simulink model "IM_Model"  (R2021a)
settings: Solver=ode23t  StartTime=0.0  StopTime=2  MaxStep=10^-5  RelTol=1e-3
InitFcn:
  | Rs=0.5968;
  | Lls=0.0003495;
  | Rr=0.6258;
  | Llr=0.005473;
  | Lm=0.0354;
  | Ls=Lls+Lm;
  | Lr=Llr+Lm;
  | J=0.05;
  | B=0.005879;
  | P=4;
libraries: spsControlledVoltageSourceLib x3, spsdq0toabcLib x2, spsAsynchronousMachineSIUnitsLib x1, mcbcontrolslib x1, spsabctodq0Lib x1, spspowerguiLib x1
settings Model: Creator=User  LastModifiedBy=User
settings SolverCC: AlgebraicLoopSolver=TrustRegion
settings DebuggingCC: SFMachineParentedDataDiag=warning

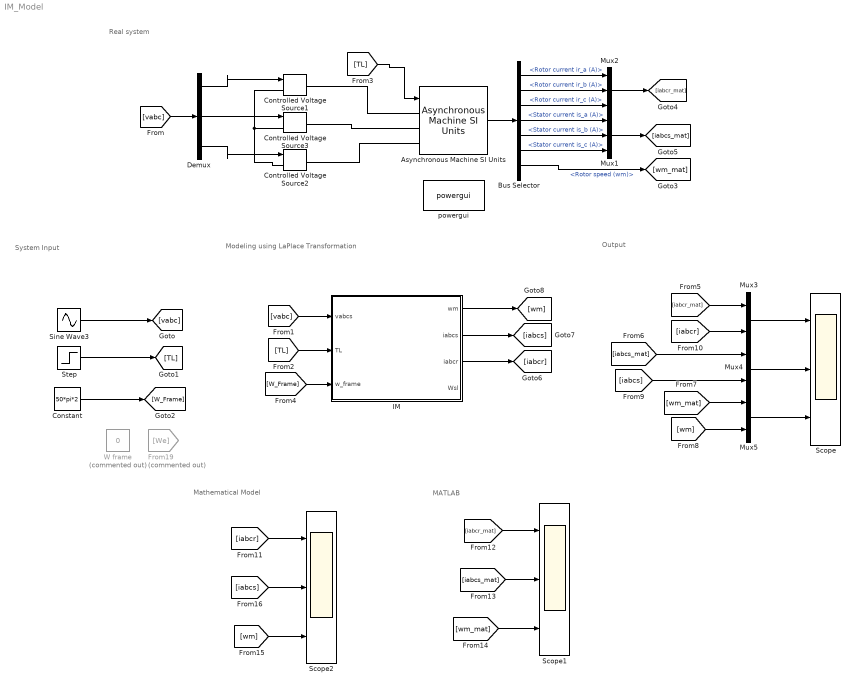
== system IM_Model ==
  note: Mathematical Model
  note: MATLAB
  note: Modeling using LaPlace Transformation
  note: Output
  note: System Input
  note: Real system
  Asynchronous Machine SI Units : spsAsynchronousMachineSIUnitsLib/Asynchronous Machine SI Units  RotorType=Squirrel-cage  PresetModel=No  MechanicalLoad=Torque Tm  ShowDetailedParameters=on  ReferenceFrame=Stationary  Units=SI  MeasurementBus=off  NominalParameters=[1e+04 400 50]  VoltageRatio=1  Stator=[Rs Lls]  Rotor=[Rr Llr]  Cage1=[0.4155 0.002066]  Cage2=[0.4168 0.0003495]  Lm=Lm  Mechanical=[J B P/2]  PolePairs=2  InitialConditions=[1 0 0 0 0 0 0 0]  SimulateSaturation=off  Saturation=[14.03593122, 27.81365428, 53.79336849, 72.68890987, 97.98006896, 148.6815601, 215.7428561, 302.9841135, 428.7778367 ; 230, 322, 414, 460, 506, 552, 598, 644, 690]  LoadFlowParameters=1492000  TsPowergui=0  TsBlock=-1  IterativeModel=Trapezoidal non iterative  IterativeDiscreteModel=Trapezoidal non iterative  Pmec=1.492e+006
  Bus Selector : BusSelector  OutputSignals=Rotor measurements.Rotor current ir_a (A),Rotor measurements.Rotor current ir_b (A),Rotor measurements.Rotor current ir_c (A),Stator measurements.Stator current is_a (A),Stator measurements.Stator current is_b (A),Stator measurements.Stator current is_c (A),Mechanical.Rotor speed (wm)
  Constant : Constant  Value=50*pi*2
  Controlled Voltage Source1 : spsControlledVoltageSourceLib/Controlled Voltage Source  Initialize=on  Source_Type=AC  Amplitude=0  Phase=0  Frequency=0  Measurements=None
  Controlled Voltage Source2 : spsControlledVoltageSourceLib/Controlled Voltage Source  Initialize=on  Source_Type=AC  Amplitude=0  Phase=0  Frequency=0  Measurements=None
  Controlled Voltage Source3 : spsControlledVoltageSourceLib/Controlled Voltage Source  Initialize=on  Source_Type=AC  Amplitude=0  Phase=0  Frequency=0  Measurements=None
  Demux : Demux  Outputs=3
  From19 : From  Commented=on  GotoTag=We
  IM : Subsystem
  Mux1 : Mux  Inputs=3
  Mux2 : Mux  Inputs=3
  Mux3 : Mux  Inputs=2
  Mux4 : Mux  Inputs=2
  Mux5 : Mux  Inputs=2
  Scope : Scope  NumInputPorts=3
  Scope1 : Scope  NumInputPorts=3
  Scope2 : Scope  NumInputPorts=3
  Sine Wave3 : Sin  Amplitude=220*sqrt(2)  Frequency=2*pi*50  Phase=[0 -2*pi/3 2*pi/3]  SampleTime=0
  Step : Step  After=30  SampleTime=0
  W frame : Constant  Commented=on  Value=0
  powergui : spspowerguiLib/powergui  Priority=1  SimulationMode=Continuous  SampleTime=50e-6  frequency=60  Iterations=50  frequencyindice=50  Pbase=100e6  ErrMax=1e-4  UnitsV=kV  UnitsW=MW  buscounter=0  FunctionMessages=off  echomessages=off  EnableUseOfTLC=off  CurrentSourceSwitches=off  DisableSnubberDevices=on  DisableRonSwitches=on  DisableVfSwitches=on  DisplayEquations=off  AutomaticDiscreteSolvers=off  SolverType=Tustin/Backward Euler (TBE)  Interpol=off  ExternalGateDelay=off  methode=off  Ts=100  x0status=blocks  SPID=on  SwTol=0  HookPort=off  NonlinearTolerance=1e-4  nMaxIteration=100  ContinueOnMaxIteration=off  RestoreLinks=warning  ResistiveCurrentMeasurement=off  Frange=[0:2:500]  Ylog=off  Xlog=on  ShowGrid=off  save=off  variable=ZData  structure=0  ZoomFFT=off  StartTime=0.0  cycles=1  DisplayStyle=1  fundamental=60  FreqAxis=off  MaxFrequency=1000  frequencyindicesteady=1  RmsSteady=1  display=off
  wires:
  Demux/1 -> Controlled Voltage Source1/1
  Demux/2 -> Controlled Voltage Source3/1
  Demux/3 -> Controlled Voltage Source2/1
  [vabc] -> Demux/1
  Sine Wave3/1 -> [vabc]
  [vabc] -> IM/1(vabcs)
  Step/1 -> [TL]
  [TL] -> IM/2(TL)
  [TL] -> Asynchronous Machine SI Units/1
  [W_Frame] -> IM/3(w_frame)
  Asynchronous Machine SI Units/1 -> Bus Selector/1
  Bus Selector/1 -> Mux2/1  "<Rotor current ir_a (A)>"
  Bus Selector/2 -> Mux2/2  "<Rotor current ir_b (A)>"
  Bus Selector/3 -> Mux2/3  "<Rotor current ir_c (A)>"
  Bus Selector/4 -> Mux1/1  "<Stator current is_a (A)>"
  Bus Selector/5 -> Mux1/2  "<Stator current is_b (A)>"
  Bus Selector/6 -> Mux1/3  "<Stator current is_c (A)>"
  Bus Selector/7 -> [wm_mat]  "<Rotor speed (wm)>"
  Mux2/1 -> [iabcr_mat]
  Mux1/1 -> [iabcs_mat]
  IM/3(iabcr) -> [iabcr]
  IM/2(iabcs) -> [iabcs]
  IM/1(wm) -> [wm]
  [iabcr_mat] -> Mux3/1
  [iabcr] -> Mux3/2
  Mux3/1 -> Scope/1
  [iabcs] -> Mux4/2
  [iabcs_mat] -> Mux4/1
  Mux4/1 -> Scope/2
  [wm] -> Mux5/2
  [wm_mat] -> Mux5/1
  Mux5/1 -> Scope/3
  [iabcr_mat] -> Scope1/1
  [iabcs_mat] -> Scope1/2
  [wm_mat] -> Scope1/3
  [iabcr] -> Scope2/1
  [wm] -> Scope2/3
  [iabcs] -> Scope2/2
  Constant/1 -> [W_Frame]
  connections:
  Controlled Voltage Source2/LConn1 -- Controlled Voltage Source1/LConn1 -- Controlled Voltage Source3/LConn1
  Controlled Voltage Source1/RConn1 -- Asynchronous Machine SI Units/LConn1
  Controlled Voltage Source3/RConn1 -- Asynchronous Machine SI Units/LConn2
  Controlled Voltage Source2/RConn1 -- Asynchronous Machine SI Units/LConn3

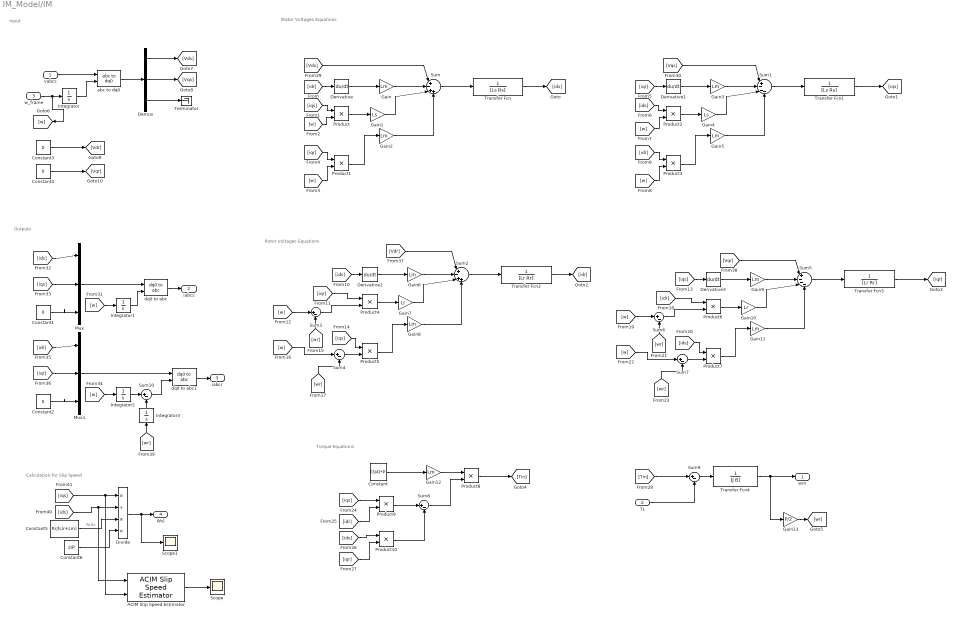
== system IM_Model/IM ==
  note: Calculation for Slip Speed
  note: Outputs
  note: Input
  note: Torque Equations
  note: Rotor Voltages Equations
  note: Stator Voltages Equations
  vabcs : Inport
  TL : Inport  Port=2
  w_frame : Inport  Port=3
  ACIM Slip Speed Estimator : mcbcontrolslib/ACIM Slip Speed Estimator  polePairs=P/2  Rr=Rr  Llr=Llr  Lm=Lm  N_sat=150  Units=Per-Unit (PU)  N_base=(120*50)/P
      settings: SourceProductBaseCode=MT
  Constant : Constant  Value=(3/4)*P  VectorParams1D=off
  Constant{1..4} (4 alike) : Constant  Value=0
  Constant5 : Constant  Value=Rr/(Llr+Lm)
  Constant6 : Constant  Value=2/P
  Demux : Demux  Outputs=3
  Derivative{,1..3} (4 alike) : Derivative
  Divide : Product  Inputs=*/**
  Gain{,2..3,5..6,8..9,11..12} (9 alike) : Gain  Gain=Lm
  Gain1 : Gain  Gain=Ls
  Gain10 : Gain  Gain=Lr
  Gain13 : Gain  Gain=P/2
  Gain4 : Gain  Gain=Ls
  Gain7 : Gain  Gain=Lr
  Integrator{,1..3} (4 alike) : Integrator
  Mux : Mux  Inputs=3
  Mux1 : Mux  Inputs=3
  Product{,1..10} (11 alike) : Product
  Scope : Scope
  Scope1 : Scope
  Sum : Sum  Inputs=|+-++
  Sum1 : Sum  Inputs=|+---
  Sum{3..4,6..10} (7 alike) : Sum  Inputs=|+-
  Sum2 : Sum  Inputs=|+-++
  Sum5 : Sum  Inputs=|+---
  Terminator : Terminator
  Transfer Fcn : TransferFcn  Denominator=[Ls Rs]
  Transfer Fcn1 : TransferFcn  Denominator=[Ls Rs]
  Transfer Fcn2 : TransferFcn  Denominator=[Lr Rr]
  Transfer Fcn3 : TransferFcn  Denominator=[Lr Rr]
  Transfer Fcn4 : TransferFcn  Denominator=[J B]
  abc to dq0 : spsabctodq0Lib/abc to dq0  Alignment=Aligned with phase A axis
  dq0 to abc : spsdq0toabcLib/dq0 to abc  Alignment=Aligned with phase A axis
  dq0 to abc1 : spsdq0toabcLib/dq0 to abc  Alignment=Aligned with phase A axis
  wm : Outport
  iabcs : Outport  Port=2
  iabcr : Outport  Port=3
  Wsl : Outport  Port=4
  wires:
  [w] -> Sum4/1
  [w] -> Product1/2
  [ids] -> Product2/1
  [wr] -> Sum4/2
  Gain8/1 -> Sum2/4
  Sum/1 -> Transfer Fcn/1
  [iqr] -> Product10/2
  Gain9/1 -> Sum5/2
  Sum2/1 -> Transfer Fcn2/1
  [iqr] -> Product4/1
  Transfer Fcn1/1 -> [iqs]
  [w] -> Product3/2
  Derivative/1 -> Gain/1
  [ids] -> Product10/1
  Sum3/1 -> Product4/2
  Derivative2/1 -> Gain6/1
  [w] -> Sum7/1
  Gain1/1 -> Sum/3
  [idr] -> Product3/1
  Gain4/1 -> Sum1/3
  [w] -> Sum6/1
  [ids] -> Product7/1
  Product3/1 -> Gain5/1
  Gain/1 -> Sum/2
  TL/1 -> Sum9/2
  Product10/1 -> Sum8/2
  [ids] -> Derivative2/1
  Gain5/1 -> Sum1/4
  Gain10/1 -> Sum5/3
  Sum8/1 -> Product8/2
  [w] -> Product2/2
  Product4/1 -> Gain7/1
  [iqr] -> Product1/1
  [iqr] -> Derivative1/1
  Product2/1 -> Gain4/1
  [w] -> Sum3/1
  [wr] -> Sum7/2
  [Vqs] -> Sum1/1
  Derivative1/1 -> Gain3/1
  Gain3/1 -> Sum1/2
  Product9/1 -> Sum8/1
  Transfer Fcn3/1 -> [iqr]
  [wr] -> Sum3/2
  [iqs] -> Product/1
  Derivative3/1 -> Gain9/1
  Product1/1 -> Gain2/1
  Sum1/1 -> Transfer Fcn1/1
  [iqs] -> Product5/1
  Product6/1 -> Gain10/1
  [idr] -> Derivative/1
  [idr] -> Product9/2
  Product5/1 -> Gain8/1
  Transfer Fcn/1 -> [ids]
  Gain2/1 -> Sum/4
  [idr] -> Product6/1
  Transfer Fcn2/1 -> [idr]
  Constant/1 -> Gain12/1
  Product/1 -> Gain1/1
  Sum4/1 -> Product5/2
  Gain6/1 -> Sum2/2
  [Vdr] -> Sum2/1
  Gain7/1 -> Sum2/3
  [iqs] -> Derivative3/1
  Gain12/1 -> Product8/1
  [iqs] -> Product9/1
  [Vqr] -> Sum5/1
  Sum5/1 -> Transfer Fcn3/1
  Sum7/1 -> Product7/2
  Product7/1 -> Gain11/1
  Gain11/1 -> Sum5/4
  [Tin] -> Sum9/1
  [wr] -> Sum6/2
  Sum6/1 -> Product6/2
  Transfer Fcn4/1 -> wm/1, Gain13/1
  Product8/1 -> [Tin]
  Sum9/1 -> Transfer Fcn4/1
  Gain13/1 -> [wr]
  abc to dq0/1 -> Demux/1
  vabcs/1 -> abc to dq0/1
  w_frame/1 -> [w], Integrator/1
  Integrator/1 -> abc to dq0/2
  [w] -> Product/2
  Demux/1 -> [Vds]
  Demux/2 -> [Vqs]
  Demux/3 -> Terminator/1
  [Vds] -> Sum/1
  Mux/1 -> dq0 to abc/1
  [w] -> Integrator1/1
  Integrator1/1 -> dq0 to abc/2
  [ids] -> Mux/1
  [iqs] -> Mux/2
  Constant1/1 -> Mux/3
  dq0 to abc/1 -> iabcs/1
  dq0 to abc1/1 -> iabcr/1
  [iqr] -> Mux1/2
  [w] -> Integrator2/1
  Constant2/1 -> Mux1/3
  Mux1/1 -> dq0 to abc1/1
  [idr] -> Mux1/1
  Constant3/1 -> [Vdr]
  Constant4/1 -> [Vqr]
  Integrator2/1 -> Sum10/1
  Sum10/1 -> dq0 to abc1/2
  Integrator3/1 -> Sum10/2
  [wr] -> Integrator3/1
  [iqs] -> ACIM Slip Speed Estimator/2, Divide/1
  [ids] -> ACIM Slip Speed Estimator/1, Divide/2
  Constant5/1 -> Divide/3  "Rr/Lr"
  Divide/1 -> Scope1/1, Wsl/1
  Constant6/1 -> Divide/4
  ACIM Slip Speed Estimator/1 -> Scope/1
